simulink model "bolusmode"  (R2023a)
settings: Solver=VariableStepAuto  StartTime=0.0  StopTime=10.0  RelTol=1e-3
settings Model: Creator=levi  LastModifiedBy=levi

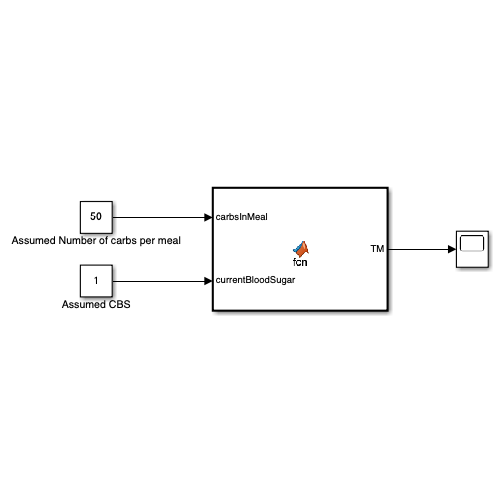
[thumbnail: Simulink's stored preview of the top-level diagram]
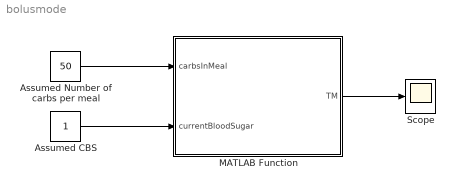
== system bolusmode ==
  Assumed CBS : Constant
  Assumed Number of carbs per meal : Constant  Value=50
  MATLAB Function : MATLAB Function  TreatAsAtomicUnit=on
  Scope : Scope
  wires:
  Assumed Number of carbs per meal/1 -> MATLAB Function/1(carbsInMeal)
  Assumed CBS/1 -> MATLAB Function/2(currentBloodSugar)
  MATLAB Function/1(TM) -> Scope/1

== matlab function bolusmode/MATLAB Function ==
  data: carbsInMeal input; currentBloodSugar input; TM output
function TM = fcn(carbsInMeal, currentBloodSugar)

  
 % Constants
    HIGH_BLOOD_SUGAR_CORRECTION_FACTOR = 1/50; % Constant for correction factor calculation
    PRE_MEAL_SUGAR_TAGET = 120;
    INSULIN_TO_CARB_RATIO = 1/10;


    %Stage 1: Carbhydrate meal coverage
    CMC = INSULIN_TO_CARB_RATIO * carbsInMeal;
    
    %Stage 2: High Sugar correction Dose;
    deltaSugar = currentBloodSugar - PRE_MEAL_SUGAR_TAGET;
    
    if deltaSugar <= 0
        CD = 0;
    else
        CD = deltaSugar * (HIGH_BLOOD_SUGAR_CORRECTION_FACTOR); 
    end
    
    %Final: Total Meal Insulin Dose
    TM = CD  + CMC
      
    


end
